simulink model "kinematics_track_Vs"  (R2021b)
settings: Solver=VariableStepAuto  StartTime=0.0  StopTime=60  RelTol=1e-10  AbsTol=1e-14
values from neighbouring files (symbols this model uses):
  q0 = [-0.8;0;pi]    [SIM01.m]    (also in SIM02.m = [j 0 the(k)]'; SIM03.m = [-1;0;-pi/2]; SIM04.m = [1 1 k]'; SIM05.m = [2;1;2])
  qr0 = [3;2;1]    [SIM05.m]
settings Model: Creator=PC  LastModifiedBy=PC
settings DataIOCC: SaveFormat=Array

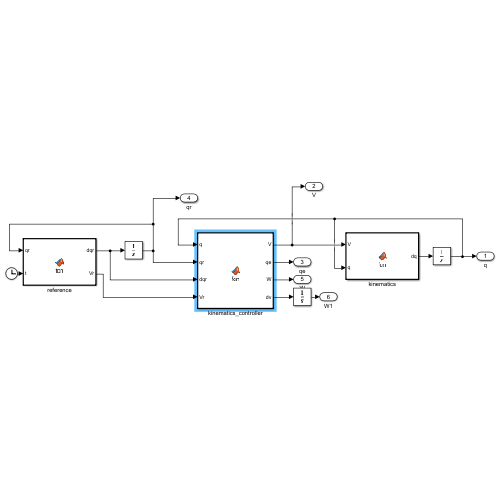
[thumbnail: Simulink's stored preview of the top-level diagram]
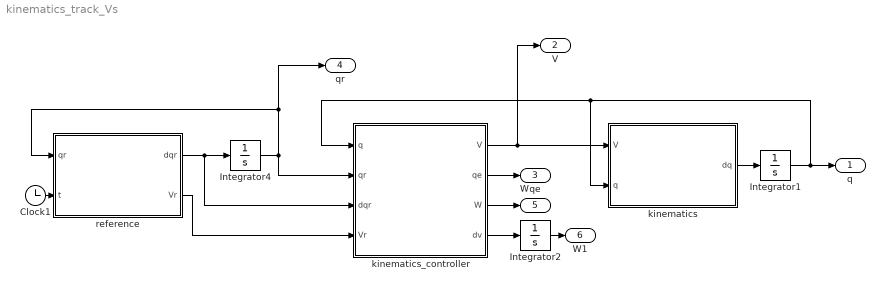
== system kinematics_track_Vs ==
  Clock1 : Clock
  Integrator1 : Integrator  InitialCondition=q0
  Integrator2 : Integrator
  Integrator4 : Integrator  InitialCondition=qr0
  kinematics : MATLAB Function  TreatAsAtomicUnit=on
  kinematics_controller : MATLAB Function  TreatAsAtomicUnit=on
  reference : MATLAB Function  TreatAsAtomicUnit=on
  q : Outport
  V : Outport  Port=2
  qe : Outport  Port=3
  qr : Outport  Port=4
  W : Outport  Port=5
  W1 : Outport  Port=6
  wires:
  kinematics_controller/2(qe) -> qe/1
  kinematics_controller/1(V) -> V/1, kinematics/1(V)
  reference/2(Vr) -> kinematics_controller/4(Vr)
  Integrator4/1 -> kinematics_controller/2(qr), reference/1(qr), qr/1
  Clock1/1 -> reference/2(t)
  reference/1(dqr) -> kinematics_controller/3(dqr), Integrator4/1
  kinematics/1(dq) -> Integrator1/1
  Integrator1/1 -> kinematics_controller/1(q), kinematics/2(q), q/1
  kinematics_controller/3(W) -> W/1
  Integrator2/1 -> W1/1
  kinematics_controller/4(dv) -> Integrator2/1

== matlab function kinematics_track_Vs/reference ==
  data: dqr output size=3*1; qr input size=3*1; Vr output size=2*1; t input
function [dqr,Vr]= fcn(qr,t)
vr=0.2;
wr=-atan(0.2*sin(0.2*t));
Vr=[vr;wr];
dqr=[cos(qr(3)) 0
     sin(qr(3)) 0
      0         1]*Vr;

== matlab function kinematics_track_Vs/kinematics_controller ==
  data: q input size=3*1; V output size=2*1; qe output size=3*1; qr input size=3*1; dqr input size=3*1; Vr input size=2*1; W output size=2*1; dv output size=1
function [V,qe,W,dv]= fcn(q,qr,dqr,Vr)
the=atan2(sin(q(3)),cos(q(3)));


k1=1;k2=3;

r=0.05;
L=0.14;
Om=10;
vm=0.5*Om*r;wm=0.5*Om*r/L;
al=atan2(dqr(2)+k1*(qr(2)-q(2)),dqr(1)+k1*(qr(1)-q(1)));
vr=Vr(1);
wr=Vr(2);
thee=atan2(sin(al-the),cos(al-the));
vp=sqrt((dqr(2)+k1*(qr(2)-q(2)))^2+(dqr(1)+k1*(qr(1)-q(1)))^2);
vd=vp*cos(thee*0.5)^2;
v=min(vd,vm);
dal=wr*vp/vr+((k1*dqr(2)-k1*v*sin(the))*cos(al)-(k1*dqr(1)-k1*v*cos(the))*sin(al))/((dqr(1)+k1*(qr(1)-q(1)))*cos(al)+(dqr(2)+k1*(qr(2)-q(2)))*sin(al));
wd=dal+2*k2*sin(thee*0.5);
w=sign(wd)*min(abs(wd),wm);
w1=v/r+L*w/r;
w2=v/r-L*w/r;
W=[w1;w2];
V=[r/2 r/2;r/(2*L) -r/(2*L)]*W;

qe=[ cos(q(3)) sin(q(3)) 0
    -sin(q(3)) cos(q(3)) 0
      0         0        1]*(qr-q);
dv=abs(V(1)-vr);

== matlab function kinematics_track_Vs/kinematics ==
  data: V input size=2*1; dq output size=3*1; q input size=3*1
function dq = fcn(V,q)
dq=[ cos(q(3))  0
     sin(q(3))  0
      0         1]*V;
